simulink model "simulink_CartpendDiscrete_KControl_neuralSensing"  (R2015a)
settings: Solver=ode45  StartTime=0.0  StopTime=20  MaxStep=0.001  RelTol=1e-3
values from neighbouring files (symbols this model uses):
  bT = 1    [run_cartSinglePendSimulink_PIDControl.m]
  bX = 1    [run_cartSinglePendSimulink_PIDControl.m]
  g = -10    [run_cartDoublePend_Control.m]    (also in run_cartSinglePendSimulink_PIDControl.m)
  K = lqr(A,B,Q,R)    [run_cartDoublePend_Control.m]    (also in run_cartSinglePendSimulink_PIDControl.m = lqr( A,B,Q,R))
  L = 2    [run_cartSinglePendSimulink_PIDControl.m]
  mc = 10    [run_cartDoublePend_Control.m]    (also in run_cartSinglePendSimulink_PIDControl.m = 5)
  mp = 1    [run_cartSinglePendSimulink_PIDControl.m]
  y0 = [0, pi, 0 ,0,0,0]    [run_cartDoublePend_Control.m]    (also in run_cartSinglePendSimulink_PIDControl.m = [-4; 0; 0; 0])
  yGoal = y0    [run_cartDoublePend_Control.m]    (also in run_cartSinglePendSimulink_PIDControl.m = y0 + [5;0;0;0])
undefined symbols (not defined in the file or in its folder): distThetaAccVariance, distXAccVariance, nDelays, neuralEncodingOn, sensorNoiseVariance, tSamp, tyGoal
libraries: simulink x4
settings Model: Creator=Thomas  LastModifiedBy=Thomas
settings DataIOCC: ExternalInput=t  InitialState=yIn  SaveState=on

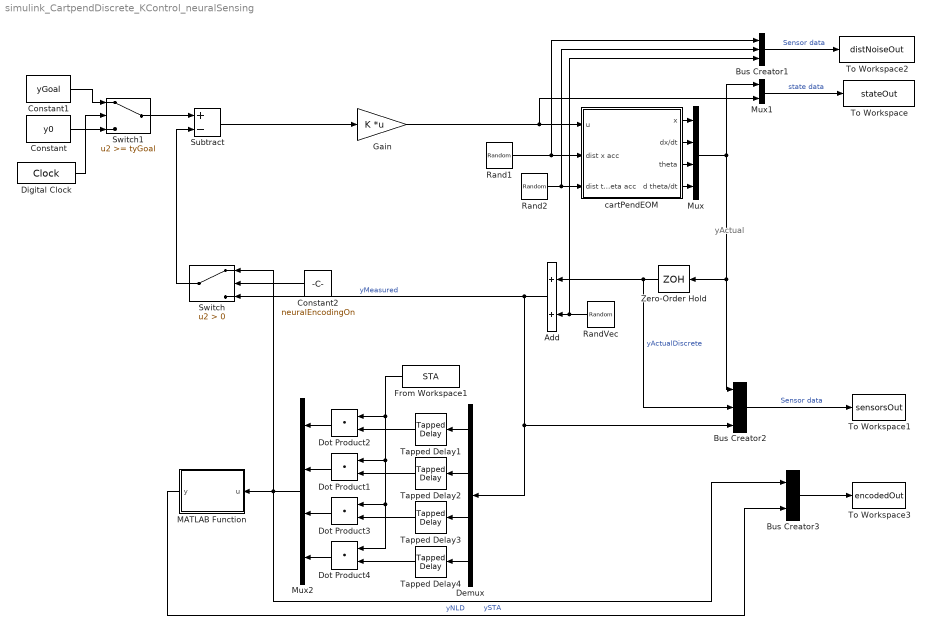
== system simulink_CartpendDiscrete_KControl_neuralSensing ==
  note: yActual
  Add : Sum
  Bus Creator1 : BusCreator  Inputs=3
  Bus Creator2 : BusCreator  Inputs=3
  Bus Creator3 : BusCreator  Inputs=2
  Constant : Constant  Value=y0  VectorParams1D=off
  Constant1 : Constant  Value=yGoal  VectorParams1D=off
  Constant2 : Constant  Value=neuralEncodingOn
  Demux : Demux
  Digital Clock : DigitalClock  SampleTime=tSamp
  Dot Product{1..4} (4 alike) : DotProduct  InputSameDT=on  OutDataTypeStr=Inherit: Inherit via internal rule
  From Workspace1 : FromWorkspace  VariableName=STA  SampleTime=tSamp
  Gain : Gain  Gain=K  Multiplication=Matrix(K*u) (u vector)
  MATLAB Function : MATLAB Function  TreatAsAtomicUnit=on
  Mux : Mux
  Mux1 : Mux  Inputs=2
  Mux2 : Mux
  Rand1 : RandomNumber  Variance=distXAccVariance  Seed=4  SampleTime=tSamp
  Rand2 : RandomNumber  Variance=distThetaAccVariance  Seed=5  SampleTime=tSamp
  RandVec : RandomNumber  Variance=sensorNoiseVariance  Seed=[0,1,2,3]  SampleTime=tSamp
  Subtract : Sum  Inputs=+-
  Switch : Switch  Criteria=u2 > Threshold
  Switch1 : Switch  Threshold=tyGoal  ZeroCross=off
  Tapped Delay1 : simulink/Discrete/Tapped Delay  vinit=y0(1)  samptime=tSamp  NumDelays=nDelays  DelayOrder=Oldest  includeCurrent=on
  Tapped Delay2 : simulink/Discrete/Tapped Delay  vinit=y0(2)  samptime=tSamp  NumDelays=nDelays  DelayOrder=Oldest  includeCurrent=on
  Tapped Delay3 : simulink/Discrete/Tapped Delay  vinit=y0(3)  samptime=tSamp  NumDelays=nDelays  DelayOrder=Oldest  includeCurrent=on
  Tapped Delay4 : simulink/Discrete/Tapped Delay  vinit=y0(4)  samptime=tSamp  NumDelays=nDelays  DelayOrder=Oldest  includeCurrent=on
  To Workspace : ToWorkspace  VariableName=stateOut  SaveFormat=Structure With Time  SampleTime=-1
  To Workspace1 : ToWorkspace  VariableName=sensorsOut  SaveFormat=Timeseries  SampleTime=-1
  To Workspace2 : ToWorkspace  VariableName=distNoiseOut  SaveFormat=Timeseries  SampleTime=-1
  To Workspace3 : ToWorkspace  VariableName=encodedOut  SaveFormat=Timeseries  SampleTime=-1
  Zero-Order Hold : ZeroOrderHold  SampleTime=tSamp
  cartPendEOM : Subsystem  mask(Inverted pendulum on cart){mc=mc, mp=mp, L=L, g=g, bX=bX, bT=bT}
      mask prompts: mc "Mass of cart (kg):"; mp "Mass of pendulum (kg):"; L "Distance to pendulum center of mass(m):"; g "Acceleration of gravity (m/s^2):"; bX "Damping of cart (kg/s)"; bT "Damping of pendulum (kg*m/s)"
      mask help: Unmask and double-click to see dynamics
      mask Help: Nonlinear dynamics of inverted pendulum on cart.
  wires:
  cartPendEOM/4(d theta/dt) -> Mux/4
  cartPendEOM/3("theta ") -> Mux/3
  cartPendEOM/2(dx/dt) -> Mux/2
  cartPendEOM/1(x) -> Mux/1
  Subtract/1 -> Gain/1
  Bus Creator2/1 -> To Workspace1/1  "Sensor data"
  Mux1/1 -> To Workspace/1  "state data"
  Mux/1 -> Bus Creator2/1, Zero-Order Hold/1, Mux1/1
  Zero-Order Hold/1 -> Add/1, Bus Creator2/2  "yActualDiscrete"
  Gain/1 -> cartPendEOM/1(u), Mux1/2
  Rand1/1 -> Bus Creator1/1, cartPendEOM/2(dist x acc)
  Rand2/1 -> Bus Creator1/2, cartPendEOM/3("dist theta acc ")
  Bus Creator1/1 -> To Workspace2/1  "Sensor data"
  RandVec/1 -> Bus Creator1/3, Add/2
  Add/1 -> Demux/1, Bus Creator2/3, Switch/3  "yMeasured"
  Demux/1 -> Tapped Delay1/1
  Tapped Delay1/1 -> Dot Product2/2
  From Workspace1/1 -> Dot Product4/1, Dot Product3/1, Dot Product1/1, Dot Product2/1
  Dot Product2/1 -> Mux2/1
  Mux2/1 -> Bus Creator3/1, Switch/1, MATLAB Function/1(u)  "ySTA"
  Demux/2 -> Tapped Delay2/1
  Demux/4 -> Tapped Delay4/1
  Demux/3 -> Tapped Delay3/1
  Tapped Delay2/1 -> Dot Product1/2
  Tapped Delay3/1 -> Dot Product3/2
  Tapped Delay4/1 -> Dot Product4/2
  Dot Product1/1 -> Mux2/2
  Dot Product3/1 -> Mux2/3
  Dot Product4/1 -> Mux2/4
  Digital Clock/1 -> Switch1/2
  Switch1/1 -> Subtract/1
  Constant/1 -> Switch1/3
  Constant1/1 -> Switch1/1
  Switch/1 -> Subtract/2
  Constant2/1 -> Switch/2
  MATLAB Function/1(y) -> Bus Creator3/2  "yNLD"
  Bus Creator3/1 -> To Workspace3/1

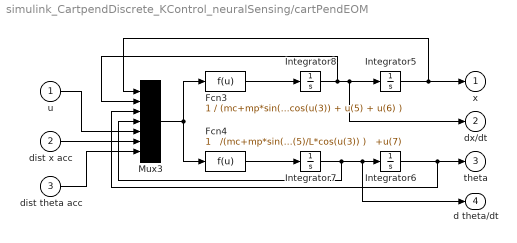
== system simulink_CartpendDiscrete_KControl_neuralSensing/cartPendEOM ==
  u : Inport
  dist x acc : Inport  Port=2
  "dist theta acc " : Inport  Port=3
  Fcn3 : Fcn  Expr="1 / (mc+mp*sin(u(3))^2)  * (   u(4)^2*mp*L*sin(u(3)) -u(4)*bT/L*cos(u(3))   -u(2)*bX  -   mp*g*sin(u(3))*cos(u(3)) + u(5) + u(6) )"
  Fcn4 : Fcn  Expr="1   /(mc+mp*sin(u(3))^2)  * (   u(2)*bX/L*cos(u(3))   -   u(4)^2*mp*sin(u(3))*cos(u(3))   - u(4)*bT*(mc+mp)/ (L^2*mp)       + (mc+mp)*g/L*sin(u(3)) - u(5)/L*cos(u(3)) )   +u(7)"
  Integrator5 : Integrator  InitialCondition=y0(1)  ContinuousStateAttributes='x'
  Integrator6 : Integrator  InitialCondition=y0(3)  ContinuousStateAttributes='theta'
  Integrator7 : Integrator  InitialCondition=y0(4)  ContinuousStateAttributes='theta_dot'
  Integrator8 : Integrator  InitialCondition=y0(2)  ContinuousStateAttributes='xDot'
  Mux3 : Mux  Inputs=7
  x : Outport  InitialOutput=0
  dx/dt : Outport  Port=2  InitialOutput=0
  "theta " : Outport  Port=3  InitialOutput=0
  d theta/dt : Outport  Port=4  InitialOutput=0
  wires:
  Integrator5/1 -> Mux3/1, x/1
  Fcn4/1 -> Integrator7/1
  Mux3/1 -> Fcn3/1, Fcn4/1
  Fcn3/1 -> Integrator8/1
  Integrator8/1 -> Mux3/2, dx/dt/1, Integrator5/1
  Integrator7/1 -> Mux3/4, d theta/dt/1, Integrator6/1
  Integrator6/1 -> Mux3/3, "theta "/1
  u/1 -> Mux3/5
  dist x acc/1 -> Mux3/6
  "dist theta acc "/1 -> Mux3/7

== matlab function simulink_CartpendDiscrete_KControl_neuralSensing/MATLAB Function ==
  data: u input; y output
function y = NLD(u)
%#codegen

NLDs = [0.5];
NLDg = [10];
y = ( 1./ (1+ exp(-NLDg.*(u-NLDs)) ) - 0.5) + 0.5;
